simulink model "linedetect_v1"  (Simulink 7.6)
settings: Solver=ode45  StartTime=0.0  StopTime=10.0  RelTol=1e-3
undefined symbols (not defined in the file): Hedge_Hue, Rec, SDTV, strel
libraries: vipconversions x5, vipsnks x4, simulink x2, viptransforms x2, vipmorphops x1, viptextngfix x1, vipanalysis x1, vipsrcs x1
settings Model: Creator=Thing 1  LastModifiedBy=Administrator

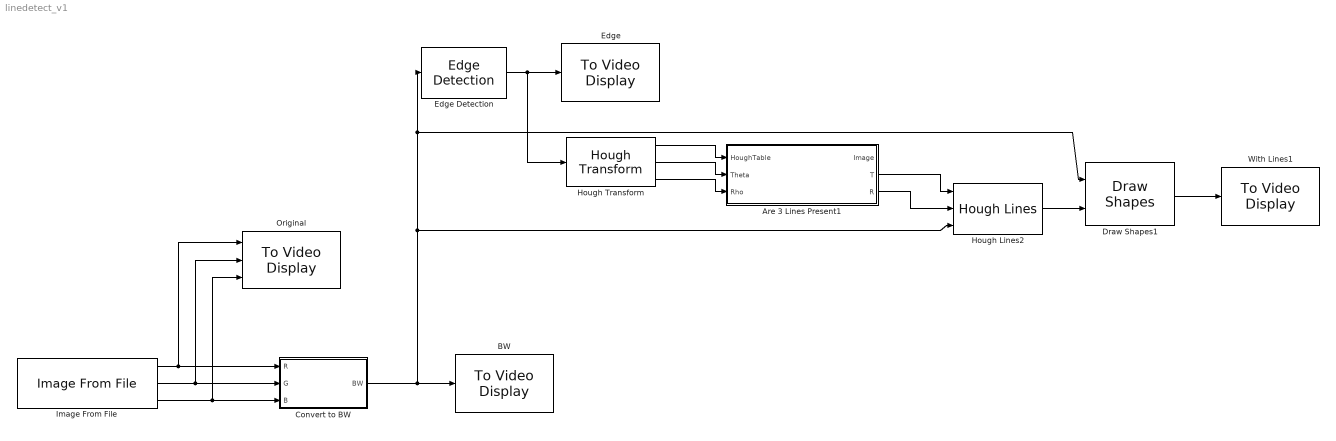
== system linedetect_v1 ==
  Are 3 Lines Present1 : Stateflow chart  TreatAsAtomicUnit=on
  BW : vipsnks/To Video Display  DialogControllerArgs=DataTag0  inputType=Obsolete  imagePorts=One multidimensional signal  OutputDevice=On-screen video monitor  fullScreen=off  videoWindowX=547  videoWindowY=21  saveWindowSize=off  videoWindowWidth=160  videoWindowHeight=120  dataOrg=Column-major  openAtMdlStart=on  isWindowOpen=on
  Convert to BW : Subsystem
  Draw Shapes1 : viptextngfix/Draw Shapes  DialogController=vipDDGCreate  DialogControllerArgs=DataTag4  shape=Lines  fill=off  fillClrSource=Specify via dialog  display=User-specified value  intensity=200  color=.8  opacity=0.6  viewport=Entire image  antialiasing=off  inType=Obsolete  imagePorts=One multidimensional signal  prodOutputMode=Binary point scaling  prodOutputWordLength=32  prodOutputFracLength=14  memoryMode=Specify word length  memoryWordLength=16  memoryFracLength=15  roundingMode=Floor  overflowMode=off
  Edge : vipsnks/To Video Display  DialogControllerArgs=DataTag5  inputType=Obsolete  imagePorts=One multidimensional signal  OutputDevice=On-screen video monitor  fullScreen=off  videoWindowX=427  videoWindowY=224  saveWindowSize=off  videoWindowWidth=160  videoWindowHeight=120  dataOrg=Column-major  openAtMdlStart=on  isWindowOpen=on
  Edge Detection : vipanalysis/Edge Detection  DialogController=vipDDGCreate  DialogControllerArgs=DataTag6  method=Sobel  outputType=Binary image  userDefinedThreshold=off  thresholdSource=Specify via dialog  threshold=20  thresholdTuning=3  edgeThinning=on  threshold_canny=[0.25 0.60]  autoPercent=70  sigma=1  roundingMode=Floor  overflowMode=off
  Hough Lines2 : viptransforms/Hough Lines  DialogController=vipDDGCreate  DialogControllerArgs=DataTag7  sineCompMethod=Trigonometric function  thetaRes=pi/180  firstCoeffMode=Specify word length  firstCoeffWordLength=16  firstCoeffFracLength=15  prodOutputMode=Binary point scaling  prodOutputWordLength=32  prodOutputFracLength=16  roundingMode=Nearest  overflowMode=on
  Hough Transform : viptransforms/Hough Transform  DialogController=vipDDGCreate  DialogControllerArgs=DataTag8  theta_res=pi/180  rho_res=1  out_theta_rho=on  outdtmode=double  firstCoeffMode=Binary point scaling  firstCoeffWordLength=16  firstCoeffFracLength=14  secondCoeffMode=Binary point scaling  secondCoeffWordLength=32  secondCoeffFracLength=16  outputMode=Binary point scaling  outputWordLength=16  outputFracLength=0  accumMode=Binary point scaling  accumWordLength=32  accumFracLength=20  prodOutputMode=Binary point scaling  prodOutputWordLength=32  prodOutputFracLength=20  memoryMode=Binary point scaling  memoryWordLength=32  memoryFracLength=16  roundingMode=Nearest  overflowMode=on
  Image From File : vipsrcs/Image From File  Tag=vipblks_nd  DialogController=vipDDGCreate  DialogControllerArgs=DataTag9  SystemSampleTime=-1  FileName=C:\Documents and Settings\Administrator\My Documents\Academics\Spring 2011\AUVT - Vision\src\vision\gate1.PNG  imagePorts=Separate color signals  Ts=1  ImageDataType=double  Signed=on  WordLength=16  sdImageDataType=uint(8)  FractionLengthMode=User-defined  FractionLength=15  OutPortLabels=R|G|B
  Original : vipsnks/To Video Display  DialogControllerArgs=DataTag10  inputType=Obsolete  imagePorts=Separate color signals  OutputDevice=On-screen video monitor  fullScreen=off  videoWindowX=74  videoWindowY=198  saveWindowSize=off  videoWindowWidth=160  videoWindowHeight=120  dataOrg=Column-major  openAtMdlStart=on  isWindowOpen=on
  With Lines1 : vipsnks/To Video Display  DialogControllerArgs=DataTag11  inputType=Obsolete  imagePorts=One multidimensional signal  OutputDevice=On-screen video monitor  fullScreen=off  videoWindowX=998  videoWindowY=339  saveWindowSize=off  videoWindowWidth=160  videoWindowHeight=120  dataOrg=Column-major  openAtMdlStart=on  isWindowOpen=on
  wires:
  Image From File/1 -> Original/1, Convert to BW/1(R)
  Image From File/2 -> Original/2, Convert to BW/2(G)
  Image From File/3 -> Original/3, Convert to BW/3(B)
  Convert to BW/1(BW) -> BW/1, Hough Lines2/3, Edge Detection/1, Draw Shapes1/1
  Edge Detection/1 -> Edge/1, Hough Transform/1
  Draw Shapes1/1 -> With Lines1/1
  Hough Transform/2 -> Are 3 Lines Present1/2(Theta)
  Hough Transform/3 -> Are 3 Lines Present1/3(Rho)
  Hough Transform/1 -> Are 3 Lines Present1/1(HoughTable)
  Are 3 Lines Present1/3(R) -> Hough Lines2/2
  Are 3 Lines Present1/2(T) -> Hough Lines2/1
  Hough Lines2/1 -> Draw Shapes1/2

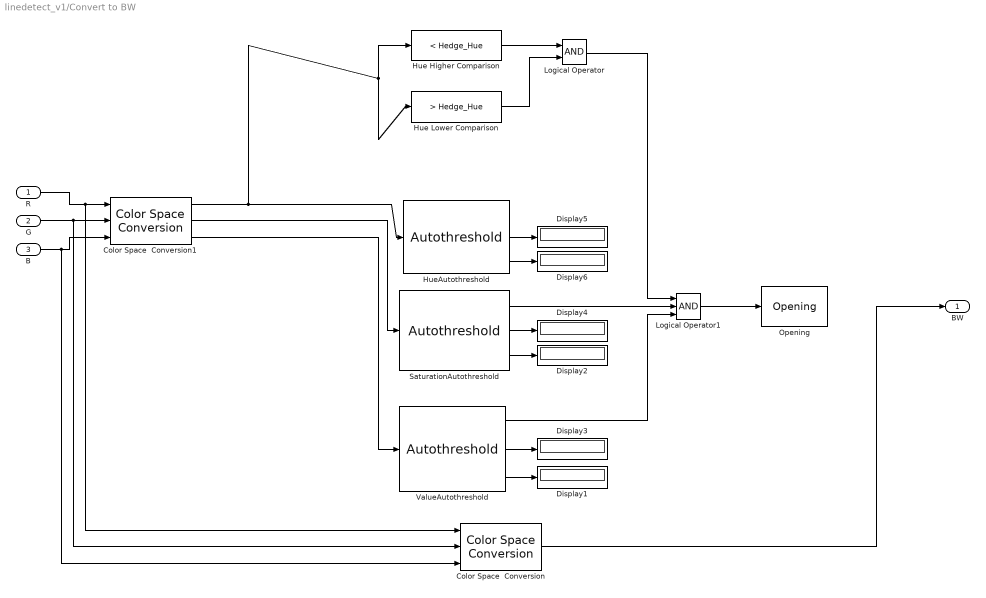
== system linedetect_v1/Convert to BW ==
  R : Inport  OutDataTypeStr=double
  G : Inport  Port=2  OutDataTypeStr=double
  B : Inport  Port=3  OutDataTypeStr=double
  Color Space  Conversion : vipconversions/Color Space  Conversion  conversion=Obsolete  conversionActive=R'G'B' to intensity  wp_str=D65  rec=Rec. 601 (SDTV)  sys=1125/60/2:1  imagePorts=Separate color signals
  Color Space  Conversion1 : vipconversions/Color Space  Conversion  conversion=Obsolete  conversionActive=R'G'B' to HSV  wp_str=D65  rec=Rec. 601 (SDTV)  sys=1125/60/2:1  imagePorts=Separate color signals
  Display{1..6} (6 alike) : Display
  Hue Higher Comparison : simulink/Logic and Bit Operations/Compare To Constant  SystemSampleTime=-1  relop=<  const=Hedge_Hue  LogicOutDataTypeMode=boolean  ZeroCross=off
  Hue Lower Comparison : simulink/Logic and Bit Operations/Compare To Constant  SystemSampleTime=-1  relop=>  const=Hedge_Hue  LogicOutDataTypeMode=boolean  ZeroCross=off
  HueAutothreshold : vipconversions/Autothreshold  DialogController=vipDDGCreate  DialogControllerArgs=DataTag1  operator=>  threshOut=on  effMetricOut=on  userDefinedRange=off  umin=0  umax=255  outOfRngOpt=Warn and saturate  scaleThreshold=off  scaleFactor=1  P1Mode=Specify word length  P1WordLength=32  P1FracLength=30  P2Mode=Specify word length  P2WordLength=32  P2FracLength=22  P3Mode=Specify word length  P3WordLength=32  P3FracLength=14  P4Mode=Binary point scaling  P4WordLength=32  P4FracLength=15  Q1Mode=Specify word length  Q1WordLength=32  Q1FracLength=16  EMMode=Specify word length  EMWordLength=16  EMFracLength=14  roundingMode=Floor  overflowMode=off
  Logical Operator : Logic  AllPortsSameDT=off  OutDataTypeStr=fixdt('boolean', 'DataTypeOverride', 'Off')
  Logical Operator1 : Logic  Inputs=3
  Opening : vipmorphops/Opening  nhoodsrc=Specify via dialog  strel=strel('disk',2)
  SaturationAutothreshold : vipconversions/Autothreshold  DialogController=vipDDGCreate  DialogControllerArgs=DataTag2  operator=>  threshOut=on  effMetricOut=on  userDefinedRange=off  umin=0  umax=255  outOfRngOpt=Warn and saturate  scaleThreshold=off  scaleFactor=1  P1Mode=Specify word length  P1WordLength=32  P1FracLength=30  P2Mode=Specify word length  P2WordLength=32  P2FracLength=22  P3Mode=Specify word length  P3WordLength=32  P3FracLength=14  P4Mode=Binary point scaling  P4WordLength=32  P4FracLength=15  Q1Mode=Specify word length  Q1WordLength=32  Q1FracLength=16  EMMode=Specify word length  EMWordLength=16  EMFracLength=14  roundingMode=Floor  overflowMode=off
  ValueAutothreshold : vipconversions/Autothreshold  DialogController=vipDDGCreate  DialogControllerArgs=DataTag3  operator=>  threshOut=on  effMetricOut=on  userDefinedRange=off  umin=0  umax=255  outOfRngOpt=Warn and saturate  scaleThreshold=off  scaleFactor=1  P1Mode=Specify word length  P1WordLength=32  P1FracLength=30  P2Mode=Specify word length  P2WordLength=32  P2FracLength=22  P3Mode=Specify word length  P3WordLength=32  P3FracLength=14  P4Mode=Binary point scaling  P4WordLength=32  P4FracLength=15  Q1Mode=Specify word length  Q1WordLength=32  Q1FracLength=16  EMMode=Specify word length  EMWordLength=16  EMFracLength=14  roundingMode=Floor  overflowMode=off
  BW : Outport
  wires:
  Color Space  Conversion1/2 -> SaturationAutothreshold/1
  Color Space  Conversion1/1 -> HueAutothreshold/1, Hue Lower Comparison/1, Hue Higher Comparison/1
  SaturationAutothreshold/3 -> Display2/1
  Logical Operator/1 -> Logical Operator1/1
  ValueAutothreshold/2 -> Display3/1
  Color Space  Conversion1/3 -> ValueAutothreshold/1
  SaturationAutothreshold/1 -> Logical Operator1/2
  ValueAutothreshold/1 -> Logical Operator1/3
  HueAutothreshold/2 -> Display5/1
  HueAutothreshold/3 -> Display6/1
  SaturationAutothreshold/2 -> Display4/1
  ValueAutothreshold/3 -> Display1/1
  R/1 -> Color Space  Conversion1/1, Color Space  Conversion/1
  G/1 -> Color Space  Conversion1/2, Color Space  Conversion/2
  B/1 -> Color Space  Conversion1/3, Color Space  Conversion/3
  Hue Higher Comparison/1 -> Logical Operator/1
  Hue Lower Comparison/1 -> Logical Operator/2
  Logical Operator1/1 -> Opening/1
  Color Space  Conversion/1 -> BW/1

== matlab function Are 3 Lines Present1 ==
  data: HoughTable input double; Image output double; T output double; Theta input double; Rho input double; R output double
function [Image,T,R] = AreLinesPresent(HoughTable,Theta,Rho)
% This function is meant to see if there are 3 lines which approximate a
% 'hedge' in the current frame

R = zeros(1,2);
T = zeros(1,2);
[rhos, thetas] = size(HoughTable);

% Find the two vetical lines
theta_0_col = floor(thetas/2);

most_votes = 0;
second_most = 0;
indexi1 = 1;
indexi2 = 1;
indexj1 = 1;
indexj2 = 1;


for i = 1:rhos
    for j = theta_0_col-5:theta_0_col+5
        if(HoughTable(i,j) > most_votes)
            %{
            if(abs(Rho(indexi1)-Rho(i)) > 20)
                second_most = HoughTable(indexi1,indexj2);
                indexi2 = indexi1;
                indexj2 = indexj1;
                R(2) = R(1);
                T(2) = T(1);
            end
            %}
            most_votes = HoughTable(i,j);
            indexi1 = i;
            indexj1 = j;
            R(1) = Rho(i);
            T(1) = Theta(j);
        %{
elseif(HoughTable(i,j) > second_most && abs(Rho(indexi1)-Rho(i)) > 20)
            second_most = HoughTable(i,j);
            indexi2 = i;
            indexj2 = j;
            R(2) = Rho(i);
            T(2) = Theta(j);
%}
        end
    end
end

% Find the horizontal line
max_votes = 0;
index = [0 0];
for i = 1:rhos
    for j = 1:10
        if(HoughTable(i,j) > max_votes)
            max_votes = HoughTable(i,j);
            index = [i,j];
            R(2) = Rho(i);
            T(2) = Theta(j);
        end
    end
    for j = thetas-10:thetas
        if(HoughTable(i,j) > max_votes)
            max_votes = HoughTable(i,j);
            index = [i,j];
            R(2) = Rho(i);
            T(2) = Theta(j);
        end
    end
end

% Find the most prominent line
top_vote = 0;
t = 0;
r = 0;
for i = 1:rhos
    for j = 1:thetas
        if(HoughTable(i,j) > top_vote)
            top_vote = HoughTable(i,j);
            t = j;
            r = i;
        end
    end
end

Image = 0;
if(top_vote*.75 < max_votes && top_vote*.3 < most_votes && top_vote*.3 < second_most)
    Image = 1;
end

cow = 1;

return
